simulink library "CustomLibrary"  (R2018a)
settings: Solver=VariableStepAuto  StartTime=0.0  StopTime=10.0  RelTol=1e-3
settings Model: Creator=jonathancoulter  LastModifiedBy=jonathancoulter

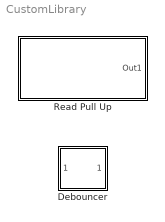
== system CustomLibrary ==
  Debouncer : Stateflow chart  TreatAsAtomicUnit=on
  Read Pull Up : Subsystem  mask{pinNumberMask=9, SampleTimeMask=0.1}
      mask prompts: pinNumberMask "Pin Number"; SampleTimeMask "Sample Time"
      mask Display:
      | pic=imread('digitalio.png');image(pic,[0.32 0.25 0.35 0.55]);text(0.5, 0.15, ['Pull Up Pin ' num2str(pinNumberMask)], 'horizontalAlignment', 'center');
      | color('blue');
      | text(0.55, 0.87, 'ARDUINO', 'horizontalAlignment', 'left');
      | color('black');

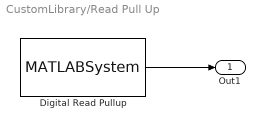
== system CustomLibrary/Read Pull Up ==
  Digital Read Pullup : MATLABSystem  System=DigitalReadPullUp  pinNumber=pinNumberMask  SampleTime=SampleTimeMask
      mask Type: DigitalReadPullUp
      mask Display:
      | disp('Digital Read PullUp');
      | port_label('output',1,'y');
  Out1 : Outport  PortDimensions=1
  wires:
  Digital Read Pullup/1 -> Out1/1

== stateflow chart CustomLibrary/Debouncer ==
  settings: sampleTime=0.001
  state Off
    en: sw_out = false;
  state Debounce
    state Off
    state On
    Debounce.Off -> Debounce.On [order 2] : [sw_in == true]
    Debounce.On -> Debounce.Off [order 2] : [sw_in == false]
  state On
    en: sw_out = true;
  (default) -> Off
  Debounce.Off -> Off [order 1] : after(100, msec)
  Off -> Debounce.On : [sw_in == true]
  Debounce.On -> On [order 1] : after(50, msec)
  On -> Debounce.Off : [sw_in == false]
  data: sw_in input; sw_out output boolean =false
